simulink model "Problrm3"  (R2020b)
settings: Solver=VariableStepAuto  StartTime=0.0  StopTime=10.0  RelTol=1e-3
values from neighbouring files (symbols this model uses):
  b = 50.0    [data.sldd]
  m = 1000.0    [data.sldd]
settings Model: DataDictionary=data.sldd  Creator=ANUJA  LastModifiedBy=ANUJA

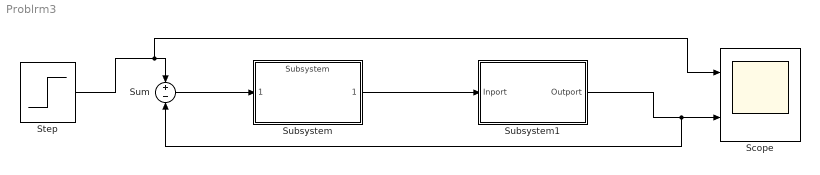
== system Problrm3 ==
  Scope : Scope  NumInputPorts=2
  Step : Step  SampleTime=0
  Subsystem : ModelReference  ModelNameDialog=Subsystem  SimulationMode=Normal  ModelReferenceVersion=1.3
  Subsystem1 : Subsystem
  Sum : Sum  Inputs=+-
  wires:
  Subsystem/1 -> Subsystem1/1(Inport)
  Step/1 -> Scope/1, Sum/1
  Subsystem1/1(Outport) -> Sum/2, Scope/2
  Sum/1 -> Subsystem/1

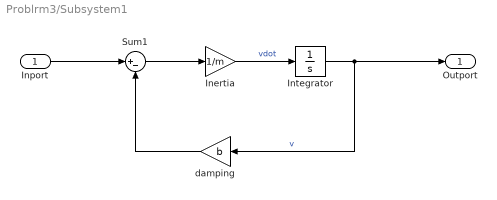
== system Problrm3/Subsystem1 ==
  Inport : Inport  OutDataTypeStr=double  PortDimensions=1  SampleTime=0
  Inertia : Gain  Gain=1/m
  Integrator : Integrator
  Sum1 : Sum  Inputs=|+-
  damping : Gain  Gain=b
  Outport : Outport  OutDataTypeStr=double  PortDimensions=1  SampleTime=0
  wires:
  Integrator/1 -> Outport/1, damping/1  "v"
  Sum1/1 -> Inertia/1
  damping/1 -> Sum1/2
  Inport/1 -> Sum1/1
  Inertia/1 -> Integrator/1  "vdot"
